simulink model "relative_orbit_prop"  (R2017b)
settings: Solver=ode4  StartTime=0.0  StopTime=stopTime  FixedStep=stepSize  RelTol=1e-3
values from neighbouring files (symbols this model uses):
  dV = [DVx;DVy;DVz]/stepSize    [AA279D_PSET2_a_change.m]
  impulseTime = 0    [AA279D_PSET2.m]    (also in AA279D_PSET2_a_change.m = tout(DVtot == min(DVtot)))
  mu = 398600    [AA279D_PSET1.m]    (also in AA279D_PSET2.m; AA279D_PSET2_a_change.m; KeplerUniversalVsSTK.m = 398600.4418; TLE_Reader.m)
  rel_pos0 = [rho_RTN_init;r0;th0]    [AA279D_PSET2.m]    (also in AA279D_PSET2_a_change.m)
  rel_vel0 = [rhod_RTN_init;rd0;thd0]    [AA279D_PSET2.m]    (also in AA279D_PSET2_a_change.m)
libraries: simulink x1
settings Model: Creator=cwcovert  LastModifiedBy=cwcovert

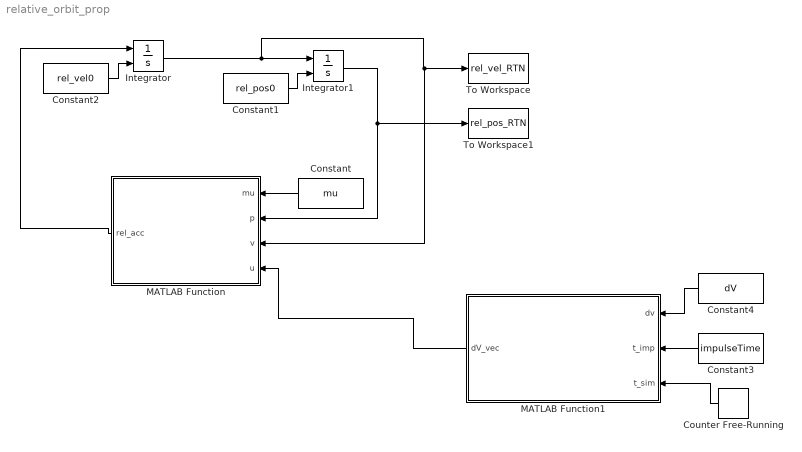
== system relative_orbit_prop ==
  Constant : Constant  Value=mu
  Constant1 : Constant  Value=rel_pos0
  Constant2 : Constant  Value=rel_vel0
  Constant3 : Constant  Value=impulseTime
  Constant4 : Constant  Value=dV
  Counter Free-Running : simulink/Sources/Counter Free-Running  NumBits=16  tsamp=stepSize
  Integrator : Integrator  InitialConditionSource=external
  Integrator1 : Integrator  InitialConditionSource=external
  MATLAB Function : MATLAB Function  TreatAsAtomicUnit=on
  MATLAB Function1 : MATLAB Function  TreatAsAtomicUnit=on
  To Workspace : ToWorkspace  VariableName=rel_vel_RTN  SampleTime=-1
  To Workspace1 : ToWorkspace  VariableName=rel_pos_RTN  SampleTime=-1
  wires:
  Constant/1 -> MATLAB Function/1(mu)
  MATLAB Function/1(rel_acc) -> Integrator/1
  Constant2/1 -> Integrator/2
  Constant1/1 -> Integrator1/2
  Integrator1/1 -> To Workspace1/1, MATLAB Function/2(p)
  Integrator/1 -> MATLAB Function/3(v), To Workspace/1, Integrator1/1
  Counter Free-Running/1 -> MATLAB Function1/3(t_sim)
  Constant4/1 -> MATLAB Function1/1(dv)
  Constant3/1 -> MATLAB Function1/2(t_imp)
  MATLAB Function1/1(dV_vec) -> MATLAB Function/4(u)

== matlab function relative_orbit_prop/MATLAB Function1 ==
  data: dv input; dV_vec output; t_imp input; t_sim input
function dV_vec = impulse_man(dv,t_imp,t_sim)

if(t_sim == t_imp)
    dV_vec = [dv(1);dv(2);dv(3);0;0];
else
    dV_vec = [0;0;0;0;0];
end

== matlab function relative_orbit_prop/MATLAB Function ==
  data: mu input; rel_acc output; p input; v input; u input
function rel_acc  = rel_accel(mu,p,v,u)

denom = ((p(4)+p(1))^2 + p(2)^2 + p(3)^2)^(3/2);

rdd = p(4)*v(5)^2 - mu/(p(4)^2)+u(4); %
thdd = -2*v(4)*v(5)/p(4)+u(5);
xdd = 2*v(5)*v(2) + thdd*p(2) + v(5)^2*p(1) -...
    (mu*(p(4)+p(1)))/denom + mu/(p(4)^2)+u(1);
ydd = -2*v(5)*v(1) - thdd*p(1) + v(5)^2*p(2) -...
    (mu*p(2))/denom+u(2);
zdd = -(mu*p(3))/denom+u(3);

rel_acc = [xdd,ydd,zdd,rdd,thdd];

end
